simulink model "ADC_model_jitter_metaestab_v2"  (R2023b)
settings: Solver=VariableStepAuto  StartTime=0.0  StopTime=simtime  FixedStep=(1/fclk)/OSR  RelTol=1e-12
model workspace (MAT data in the model file):
  Delay_242 = [0 0 0]
  ENOB_242 = -inf
  FUNDF_242 = [nan nan]
  FUNDX_242 = [-inf -inf]
  GainError_249 = [1.75 0.02734375 2.734375]
  IMODF_242 = [nan nan]
  IMODX_242 = [nan nan]
  NoiseFloor_242 = -54.2607794062
  OIP3_242 = nan
  OffsetError_249 = [0.74921875 0.0117065429687 1.17065429687]
  SFDR_242 = inf
  SINAD_242 = -inf
  SNR_242 = -inf
  THD_242 = nan
  best_linear_fit_249 = [0.0225228416502 0.00504547332987]
  bf_dnl_249 = [0.503760731487 -0.129615618295 -0.129615618295 0.0703843817053 -0.0296156182947 -0.279615618295 0.220384381705 -0.129615618295 -0.0296156182947 0.220384381705 -0.0796156182947 -0.129615618295 -0.0296156182947 -0.129615618295 0.0703843817053 -0.0296156182947 0.170384381705 -0.229615618295 -0.0296156182947 -0.0796156182947 0.220384381705 -0.129615618295 -0.129615618295 0.0703843817053 -0.129615618295 0.170384381705 -0.0296156182947 -0.129615618295 0.0703843817053 -0.0296156182947 0.170384381705 -0.179615618295 -0.0296156182947 0.0203843817053 -0.0296156182947 -0.0296156182947 0.0703843817053 0.170384381705 0.0203843817053 -0.129615618295 0.170384381705 -0.279615618295 0.0703843817053 0.170384381705 -0.179615618295 0.120384381705 0.170384381705 -0.129615618295 -0.0296156182947 0.0703843817053 0.0703843817053 -0.129615618295 0.370384381705 -0.229615618295 0.270384381705 -0.379615618295 0.420384381705 -0.0296156182947 -0.229615618295 0.170384381705 0.0703843817053 0.170384381705 -0.0796156182947 0]
  bf_inl_249 = [0 0.503760731487 0.374145113192 0.244529494898 0.314913876603 0.285298258308 0.00568264001369 0.226067021719 0.0964514034243 0.0668357851297 0.287220166835 0.20760454854 0.0779889302457 0.048373311951 -0.0812423063437 -0.0108579246384 -0.040473542933 0.129910838772 -0.0997047795224 -0.129320397817 -0.208936016112 0.0114483655936 -0.118167252701 -0.247782870996 -0.17739848929 -0.307014107585 -0.13662972588 -0.166245344174 -0.295860962469 -0.225476580764 -0.255092199058 -0.0847078173531 -0.264323435648 -0.293939053942 -0.273554672237 -0.303170290532 -0.332785908826 -0.262401527121 -0.0920171454158 -0.0716327637105 -0.201248382005 -0.0308640002998 -0.310479618594 -0.240095236889 -0.0697108551838 -0.249326473478 -0.128942091773 0.0414422899322 -0.0881733283625 -0.117788946657 -0.0474045649518 0.0229798167535 -0.106635801541 0.263748580164 0.0341329618695 0.304517343575 -0.0750982747199 0.345286106985 0.315670488691 0.0860548703961 0.256439252101 0.326823633807 0.497208015512 0.417592397217]
  delay_242 = [0 0 0]
  ep_dnl_249 = [-8.24737104007e-15 -0.128225806452 -0.128225806452 0.0717741935484 -0.0282258064516 -0.278225806452 0.221774193548 -0.128225806452 -0.0282258064516 0.221774193548 -0.0782258064516 -0.128225806452 -0.0282258064516 -0.128225806452 0.0717741935484 -0.0282258064516 0.171774193548 -0.228225806452 -0.0282258064516 -0.0782258064516 0.221774193548 -0.128225806452 -0.128225806452 0.0717741935484 -0.128225806452 0.171774193548 -0.0282258064516 -0.128225806452 0.0717741935484 -0.0282258064516 0.171774193548 -0.178225806452 -0.0282258064516 0.0217741935484 -0.0282258064516 -0.0282258064516 0.0717741935484 0.171774193548 0.0217741935484 -0.128225806452 0.171774193548 -0.278225806452 0.0717741935484 0.171774193548 -0.178225806452 0.121774193548 0.171774193548 -0.128225806452 -0.0282258064516 0.0717741935484 0.0717741935484 -0.128225806452 0.371774193548 -0.228225806452 0.271774193548 -0.378225806452 0.421774193548 -0.0282258064516 -0.228225806452 0.171774193548 0.0717741935484 0.171774193548 -0.0782258064516 0]
  ep_inl_249 = [0 -8.24737104007e-15 -0.128225806452 -0.256451612903 -0.184677419355 -0.212903225806 -0.491129032258 -0.26935483871 -0.397580645161 -0.425806451613 -0.204032258065 -0.282258064516 -0.410483870968 -0.438709677419 -0.566935483871 -0.495161290323 -0.523387096774 -0.351612903226 -0.579838709677 -0.608064516129 -0.686290322581 -0.464516129032 -0.592741935484 -0.720967741935 -0.649193548387 -0.777419354839 -0.60564516129 -0.633870967742 -0.762096774194 -0.690322580645 -0.718548387097 -0.546774193548 -0.725 -0.753225806452 -0.731451612903 -0.759677419355 -0.787903225806 -0.716129032258 -0.54435483871 -0.522580645161 -0.650806451613 -0.479032258065 -0.757258064516 -0.685483870968 -0.513709677419 -0.691935483871 -0.570161290323 -0.398387096774 -0.526612903226 -0.554838709677 -0.483064516129 -0.411290322581 -0.539516129032 -0.167741935484 -0.395967741936 -0.124193548387 -0.502419354839 -0.0806451612903 -0.108870967742 -0.337096774194 -0.165322580645 -0.0935483870968 0.0782258064516 -2.03012210217e-14]
  nbits_249 = 6
  tcr_249(1).analog = [0.00435791015625 0.0262329101562]
  tcr_249(1).digital = 0
  tcr_249(2).analog = [0.0284204101562 0.0437329101562]
  tcr_249(2).digital = 1
  tcr_249(3).analog = [0.0502954101562 0.0634204101562]
  tcr_249(3).digital = 2
  tcr_249(4).analog = [0.0699829101562 0.0896704101562]
  tcr_249(4).digital = 3
  tcr_249(5).analog = [0.0918579101562 0.107170410156]
  tcr_249(5).digital = 4
  tcr_249(6).analog = [0.118107910156 0.124670410156]
  tcr_249(6).digital = 5
  tcr_249(7).analog = [0.133420410156 0.155295410156]
  tcr_249(7).digital = 6
  tcr_249(8).analog = [0.157482910156 0.174982910156]
  tcr_249(8).digital = 7
  tcr_249(9).analog = [0.177170410156 0.190295410156]
  tcr_249(9).digital = 8
  tcr_249(10).analog = [0.205607910156 0.218732910156]
  tcr_249(10).digital = 9
  tcr_249(11).analog = [0.231857910156 0.240607910156]
  tcr_249(11).digital = 10
  tcr_249(12).analog = [0.251545410156 0.264670410156]
  tcr_249(12).digital = 11
  tcr_249(13).analog = [0.266857910156 0.286545410156]
  tcr_249(13).digital = 12
  tcr_249(14).analog = [0.288732910156 0.306232910156]
  tcr_249(14).digital = 13
  tcr_249(15).analog = [0.308420410156 0.330295410156]
  tcr_249(15).digital = 14
  tcr_249(16).analog = [0.332482910156 0.349982910156]
  tcr_249(16).digital = 15
  tcr_249(17).analog = [0.356545410156 0.378420410156]
  tcr_249(17).digital = 16
  tcr_249(18).analog = [0.380607910156 0.393732910156]
  tcr_249(18).digital = 17
  tcr_249(19).analog = [0.400295410156 0.417795410156]
  tcr_249(19).digital = 18
  tcr_249(20).analog = [0.419982910156 0.433107910156]
  tcr_249(20).digital = 19
  tcr_249(21).analog = [0.446232910156 0.465920410156]
  tcr_249(21).digital = 20
  tcr_249(22).analog = [0.468107910156 0.485607910156]
  tcr_249(22).digital = 21
  tcr_249(23).analog = [0.487795410156 0.505295410156]
  tcr_249(23).digital = 22
  tcr_249(24).analog = [0.507482910156 0.524982910156]
  tcr_249(24).digital = 23
  tcr_249(25).analog = [0.535920410156 0.549045410156]
  tcr_249(25).digital = 24
  tcr_249(26).analog = [0.551232910156 0.575295410156]
  tcr_249(26).digital = 25
  tcr_249(27).analog = [0.577482910156 0.592795410156]
  tcr_249(27).digital = 26
  tcr_249(28).analog = [0.603732910156 0.616857910156]
  tcr_249(28).digital = 27
  tcr_249(29).analog = [0.619045410156 0.638732910156]
  tcr_249(29).digital = 28
  tcr_249(30).analog = [0.645295410156 0.662795410156]
  tcr_249(30).digital = 29
  tcr_249(31).analog = [0.664982910156 0.689045410156]
  tcr_249(31).digital = 30
  tcr_249(32).analog = [0.691232910156 0.702170410156]
  tcr_249(32).digital = 31
  tcr_249(33).analog = [0.715295410156 0.724045410156]
  tcr_249(33).digital = 32
  tcr_249(34).analog = [0.737170410156 0.750295410156]
  tcr_249(34).digital = 33
  tcr_249(35).analog = [0.756857910156 0.769982910156]
  tcr_249(35).digital = 34
  tcr_249(36).analog = [0.780920410156 0.796232910156]
  tcr_249(36).digital = 35
  tcr_249(37).analog = [0.798420410156 0.820295410156]
  tcr_249(37).digital = 36
  tcr_249(38).analog = [0.822482910156 0.846545410156]
  tcr_249(38).digital = 37
  tcr_249(39).analog = [0.848732910156 0.866232910156]
  tcr_249(39).digital = 38
  tcr_249(40).analog = [0.874982910156 0.883732910156]
  tcr_249(40).digital = 39
  tcr_249(41).analog = [0.896857910156 0.912170410156]
  tcr_249(41).digital = 40
  tcr_249(42).analog = [0.920920410156 0.931857910156]
  tcr_249(42).digital = 41
  tcr_249(43).analog = [0.934045410156 0.953732910156]
  tcr_249(43).digital = 42
  tcr_249(44).analog = [0.960295410156 0.982170410156]
  tcr_249(44).digital = 43
  tcr_249(45).analog = [0.984357910156 0.997482910156]
  tcr_249(45).digital = 44
  tcr_249(46).analog = [1.00623291016 1.02373291016]
  tcr_249(46).digital = 45
  tcr_249(47).analog = [1.03029541016 1.05217041016]
  tcr_249(47).digital = 46
  tcr_249(48).analog = [1.05435791016 1.06967041016]
  tcr_249(48).digital = 47
  tcr_249(49).analog = [1.07623291016 1.08935791016]
  tcr_249(49).digital = 48
  tcr_249(50).analog = [1.10029541016 1.11779541016]
  tcr_249(50).digital = 49
  tcr_249(51).analog = [1.11998291016 1.13967041016]
  tcr_249(51).digital = 50
  tcr_249(52).analog = [1.14623291016 1.15935791016]
  tcr_249(52).digital = 51
  tcr_249(53).analog = [1.16592041016 1.19217041016]
  tcr_249(53).digital = 52
  tcr_249(54).analog = [1.19435791016 1.20967041016]
  tcr_249(54).digital = 53
  tcr_249(55).analog = [1.21185791016 1.23810791016]
  tcr_249(55).digital = 54
  tcr_249(56).analog = [1.24029541016 1.24904541016]
  tcr_249(56).digital = 55
  tcr_249(57).analog = [1.25779541016 1.27967041016]
  tcr_249(57).digital = 56
  tcr_249(58).analog = [1.29060791016 1.30592041016]
  tcr_249(58).digital = 57
  tcr_249(59).analog = [1.30810791016 1.32123291016]
  tcr_249(59).digital = 58
  tcr_249(60).analog = [1.32779541016 1.34748291016]
  tcr_249(60).digital = 59
  tcr_249(61).analog = [1.35404541016 1.37154541016]
  tcr_249(61).digital = 60
  tcr_249(62).analog = [1.37810791016 1.39998291016]
  tcr_249(62).digital = 61
  tcr_249(63).analog = [1.40217041016 1.41529541016]
  tcr_249(63).digital = 62
  tcr_249(64).analog = [1.42842041016 1.74998291016]
  tcr_249(64).digital = 63
  v_high_249 = 1.4
  v_low_249 = 0
values from neighbouring files (symbols this model uses):
  Ah2 = 0    [dynamic_charac_defaultvalues.mat]    (also in static_charac_defaultvalues.mat = 4.24264068712e-05)
  Ah3 = 0    [dynamic_charac_defaultvalues.mat]    (also in static_charac_defaultvalues.mat = 0.000707106781187)
  Ah4 = 0    [dynamic_charac_defaultvalues.mat]    (also in static_charac_defaultvalues.mat = 4.24264068712e-05)
  Ah5 = 0    [dynamic_charac_defaultvalues.mat]    (also in static_charac_defaultvalues.mat = 0.000141421356237)
  Ain = 0.45    [dynamic_charac_defaultvalues.mat]    (also in static_charac_defaultvalues.mat)
  B = 8    [dynamic_charac_defaultvalues.mat]    (also in static_charac_defaultvalues.mat)
  clock_type = 2    [dynamic_charac_defaultvalues.mat]    (also in static_charac_defaultvalues.mat)
  comparator_noise_state = 1    [dynamic_charac_defaultvalues.mat]    (also in static_charac_defaultvalues.mat)
  const = 0.8    [dynamic_charac_defaultvalues.mat]    (also in static_charac_defaultvalues.mat)
  e1 = 0    [dynamic_charac_defaultvalues.mat]    (also in static_charac_defaultvalues.mat)
  e2 = 0    [dynamic_charac_defaultvalues.mat]    (also in static_charac_defaultvalues.mat)
  e3 = 0    [dynamic_charac_defaultvalues.mat]    (also in static_charac_defaultvalues.mat)
  eoff = 0    [dynamic_charac_defaultvalues.mat]    (also in static_charac_defaultvalues.mat)
  fclk = 100000000    [dynamic_charac_defaultvalues.mat]    (also in static_charac_defaultvalues.mat)
  fin = 38337.7075195    [dynamic_charac_defaultvalues.mat]    (also in static_charac_defaultvalues.mat = 1)
  final_value = 1.25    [dynamic_charac_defaultvalues.mat]    (also in static_charac_defaultvalues.mat)
  FS = 1    [dynamic_charac_defaultvalues.mat]    (also in static_charac_defaultvalues.mat)
  fs = 390625    [dynamic_charac_defaultvalues.mat]    (also in static_charac_defaultvalues.mat = 1)
  initial_value = 0    [dynamic_charac_defaultvalues.mat]    (also in static_charac_defaultvalues.mat)
  input_type = 3    [dynamic_charac_defaultvalues.mat]    (also in static_charac_defaultvalues.mat = 1)
  M = 1280    [dynamic_charac_defaultvalues.mat]    (also in static_charac_defaultvalues.mat)
  mean_alpha = 0    [dynamic_charac_defaultvalues.mat]    (also in static_charac_defaultvalues.mat)
  mean_beta = 0.5    [dynamic_charac_defaultvalues.mat]    (also in static_charac_defaultvalues.mat)
  noise_Vrms = 0.0001    [dynamic_charac_defaultvalues.mat]    (also in static_charac_defaultvalues.mat)
  OSR = 2    [dynamic_charac_defaultvalues.mat]    (also in static_charac_defaultvalues.mat)
  ramp_noise_state = 1    [dynamic_charac_defaultvalues.mat]    (also in static_charac_defaultvalues.mat)
  SEED1 = 15581    [dynamic_charac_defaultvalues.mat]    (also in static_charac_defaultvalues.mat = 13575)
  SEED2 = 7150    [dynamic_charac_defaultvalues.mat]    (also in static_charac_defaultvalues.mat = 7577)
  sigma_alpha = 1e-10    [dynamic_charac_defaultvalues.mat]    (also in static_charac_defaultvalues.mat)
  sigma_beta = 1e-10    [dynamic_charac_defaultvalues.mat]    (also in static_charac_defaultvalues.mat)
  tau = 1e-16    [dynamic_charac_defaultvalues.mat]    (also in static_charac_defaultvalues.mat = 1e-11)
  tphase = 1e-08    [dynamic_charac_defaultvalues.mat]    (also in static_charac_defaultvalues.mat)
  Ts = 1e-08    [dynamic_charac_defaultvalues.mat]    (also in static_charac_defaultvalues.mat)
  Vnoise_comparator = 1e-10    [dynamic_charac_defaultvalues.mat]    (also in static_charac_defaultvalues.mat)
  Vnoise_ramp = 1e-10    [dynamic_charac_defaultvalues.mat]    (also in static_charac_defaultvalues.mat)
  Vof_comparator = 0    [dynamic_charac_defaultvalues.mat]    (also in static_charac_defaultvalues.mat)
libraries: simulink x4, simulink_extras x2, msbAdcFoundation x1
settings Model: SimulationMode=accelerator  Creator=mario  LastModifiedBy=mario
settings SolverCC: ZeroCrossAlgorithm=Adaptive
settings DataIOCC: SaveOutput=off  SignalLogging=off  DSMLogging=off  SaveTime=off

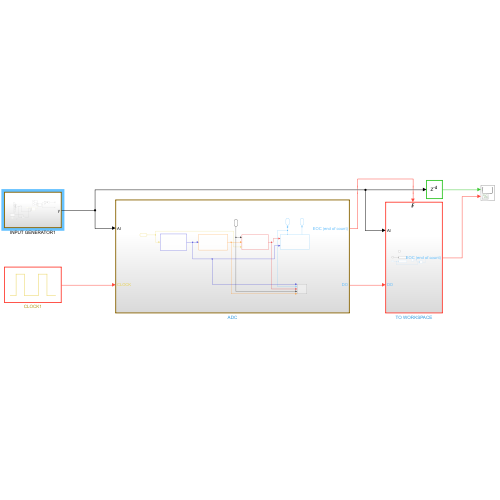
[thumbnail: Simulink's stored preview of the top-level diagram]
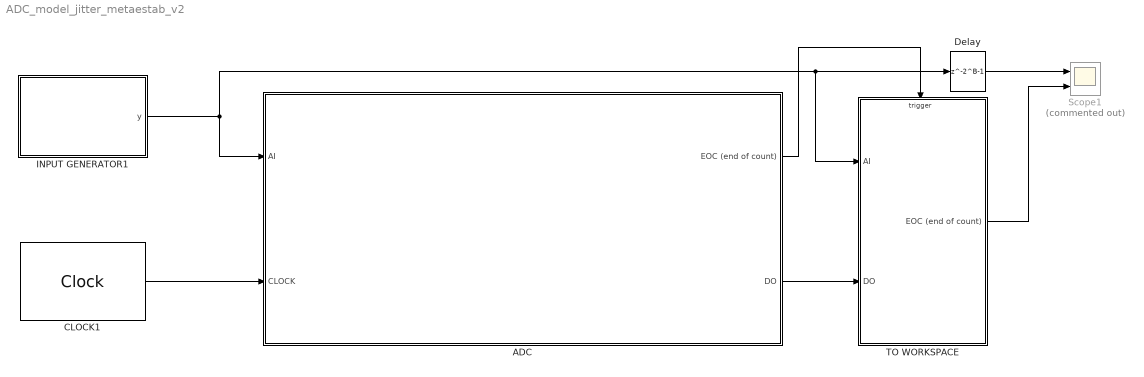
== system ADC_model_jitter_metaestab_v2 ==
  ADC : Subsystem
  CLOCK1 : simulink_extras/Flip Flops/Clock  period=1/fclk
  Delay : Delay  DelayLength=2^B-1  InitialCondition=0  SampleTime=1/fclk
  INPUT GENERATOR1 : Subsystem
  Scope1 : Scope  Commented=on  NumInputPorts=2
  TO WORKSPACE : Subsystem
  wires:
  ADC/1(EOC (end of count)) -> TO WORKSPACE/Trigger
  INPUT GENERATOR1/1(y) -> ADC/1(AI), TO WORKSPACE/1(AI), Delay/1
  TO WORKSPACE/1(EOC (end of count)) -> Scope1/2
  Delay/1 -> Scope1/1
  CLOCK1/1 -> ADC/2(CLOCK)
  ADC/2(DO) -> TO WORKSPACE/2(DO)

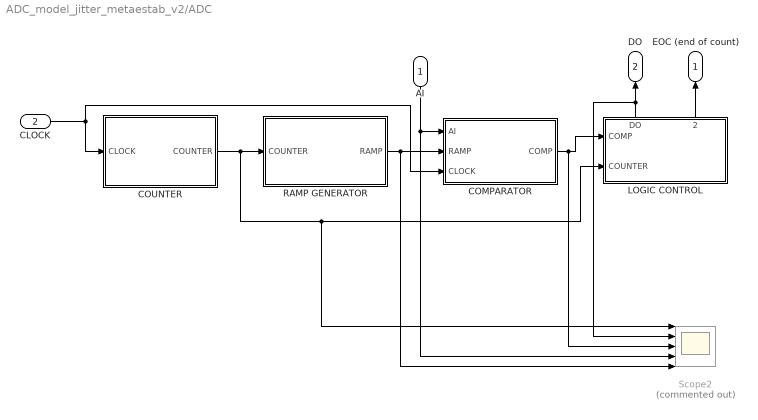
== system ADC_model_jitter_metaestab_v2/ADC ==
  AI : Inport
  CLOCK : Inport  Port=2
  COMPARATOR : Subsystem
  COUNTER : Subsystem
  LOGIC CONTROL : Subsystem
      settings: PortSchema="{\"entries\":[{\"content\":{\"sides\":[{\"content\":{},\"type\":\"ConnectorPlacement.EquallySpacedRectSide\",\"uuid\":\"4dac15f4-60b2-47ff-be01-608d4a6ba830\"},{\"content\":{\"connectorIds\":[\"Out1\",\"Out2\"],\"side\":\"RIGHT\"},\"type\":\"ConnectorPlacement.EquallySpacedRectSide\",\"uuid\":\"a37273df-03c3-4eb4-bc46-6efba4b33bab\"},{\"content\":{\"connectorIds\":[\"In1\",\"In2\"],\"side\":\"TOP\"},\"type\":\"ConnectorPlacement.EquallySpacedRectSide\",\"uuid\":\"d6687def-ae8a-4e2e-b37c-f0a7dff58a2e\"}]},\"type\":\"ConnectorPlacement.EquallySpacedConnector\",\"uuid\":\"dcf8488a-4d66-42cb-896c-32122c97ab88\"}],\"packageUris\":[\"http://schema.mathworks.com/mf0/Connector/R2020b\"],\"version\":\"1.0\"}"
  RAMP GENERATOR : Subsystem
  Scope2 : Scope  Commented=on  NumInputPorts=5
  EOC (end of count) : Outport
  DO : Outport  Port=2
  wires:
  CLOCK/1 -> COMPARATOR/3(CLOCK), COUNTER/1(CLOCK)
  AI/1 -> Scope2/4, COMPARATOR/1(AI)
  LOGIC CONTROL/1(DO) -> Scope2/2, DO/1
  LOGIC CONTROL/2(EOC (end of count)) -> EOC (end of count)/1
  COMPARATOR/1(COMP) -> Scope2/3, LOGIC CONTROL/2(COMP)
  COUNTER/1(COUNTER) -> Scope2/1, LOGIC CONTROL/1(COUNTER), RAMP GENERATOR/1(COUNTER)
  RAMP GENERATOR/1(RAMP) -> Scope2/5, COMPARATOR/2(RAMP)

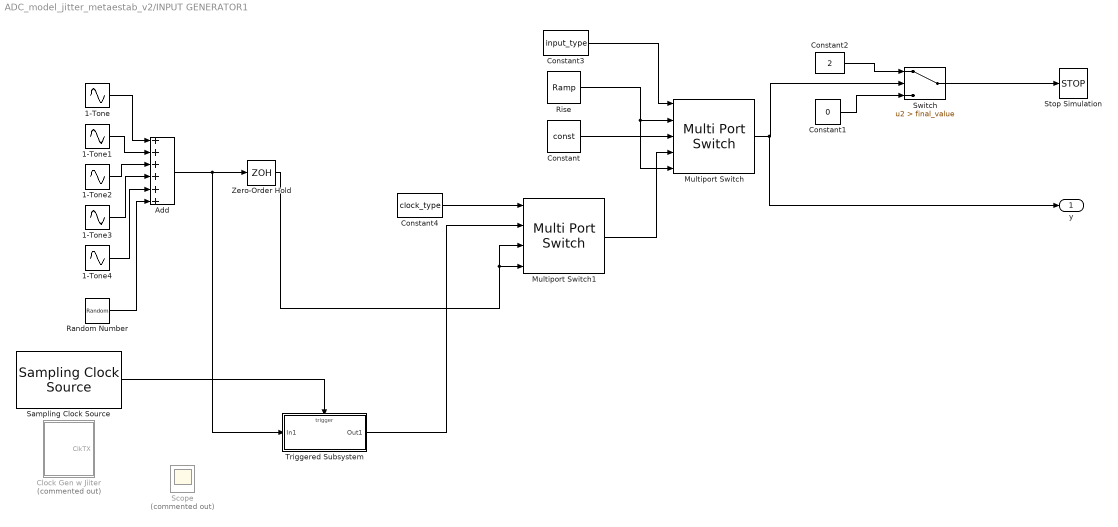
== system ADC_model_jitter_metaestab_v2/INPUT GENERATOR1 ==
  1-Tone : Sin  Amplitude=Ain  Bias=FS/2  Frequency=2 * pi * fin  SampleTime=0
  1-Tone1 : Sin  Amplitude=Ah2  Frequency=2 * pi * 2*fin  Phase=2*pi*randn  SampleTime=0
  1-Tone2 : Sin  Amplitude=Ah3  Frequency=2 * pi * 3*fin  Phase=2*pi*randn  SampleTime=0
  1-Tone3 : Sin  Amplitude=Ah4  Frequency=2 * pi * 4*fin  Phase=2*pi*randn  SampleTime=0
  1-Tone4 : Sin  Amplitude=Ah5  Frequency=2 * pi * 5*fin  Phase=2*pi*randn  SampleTime=0
  Add : Sum  Inputs=++++++
  Clock Gen w Jiiter : Subsystem  Commented=on
  Constant : Constant  Value=const
  Constant1 : Constant  Value=0
  Constant2 : Constant  Value=2
  Constant3 : Constant  Value=input_type
  Constant4 : Constant  Value=clock_type
  Multiport Switch : MultiPortSwitch  DataPortForDefault=Additional data port  DiagnosticForDefault=None  SaturateOnIntegerOverflow=off  InputSameDT=off
  Multiport Switch1 : MultiPortSwitch  Inputs=2  DataPortForDefault=Additional data port  DiagnosticForDefault=None  SaturateOnIntegerOverflow=off  InputSameDT=off
  Random Number : RandomNumber  Variance=noise_Vrms^2  SampleTime=0
  Rise : simulink/Sources/Ramp  slope=FS/((1/fclk)*(2^B)*(M))  start=0  InitialOutput=initial_value
  Sampling Clock Source : msbAdcFoundation/Sampling Clock Source  Freq=fs  Min=0  Max=1  RmsJitt=ap_jitter  CustomSeed=off  Seed=0  CustomInitialOutput=off  InitialOutput=1  ExtraBuffer=off  NBuffer=50
      settings: SignalType=Square wave
  Scope : Scope  Commented=on  NumInputPorts=2
  Stop Simulation : Stop
  Switch : Switch  Criteria=u2 > Threshold  Threshold=final_value  SaturateOnIntegerOverflow=off  InputSameDT=off
  Triggered Subsystem : Subsystem  TreatAsAtomicUnit=on
  Zero-Order Hold : ZeroOrderHold  SampleTime=1/fs
  y : Outport
  wires:
  Zero-Order Hold/1 -> Multiport Switch1/3, Multiport Switch1/4
  1-Tone/1 -> Add/1
  1-Tone1/1 -> Add/2
  Random Number/1 -> Add/6
  1-Tone4/1 -> Add/5
  1-Tone3/1 -> Add/4
  1-Tone2/1 -> Add/3
  Add/1 -> Triggered Subsystem/1(In1), Zero-Order Hold/1
  Constant4/1 -> Multiport Switch1/1
  Triggered Subsystem/1(Out1) -> Multiport Switch1/2
  Multiport Switch1/1 -> Multiport Switch/4
  Multiport Switch/1 -> Switch/2, y/1
  Rise/1 -> Multiport Switch/5, Multiport Switch/2
  Constant3/1 -> Multiport Switch/1
  Constant/1 -> Multiport Switch/3
  Switch/1 -> Stop Simulation/1
  Constant1/1 -> Switch/3
  Constant2/1 -> Switch/1
  Sampling Clock Source/1 -> Triggered Subsystem/Trigger

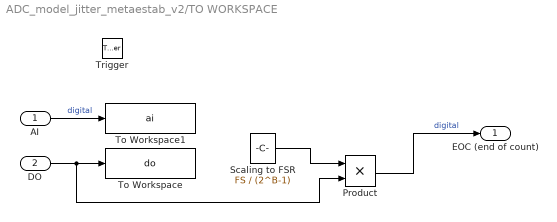
== system ADC_model_jitter_metaestab_v2/TO WORKSPACE ==
  AI : Inport
  DO : Inport  Port=2
  Trigger : TriggerPort  VariantControl=Variant  ZeroCross=off  PortDimensions=1
  Product : Product
  Scaling to FSR : Constant  Value=FS / (2^B-1)
  To Workspace : ToWorkspace  VariableName=do  SaveFormat=Structure With Time  SampleTime=-1
      settings: Save2DSignal=2-D array (concatenate along first dimension)
  To Workspace1 : ToWorkspace  VariableName=ai  SaveFormat=Structure  SampleTime=-1
      settings: Save2DSignal=2-D array (concatenate along first dimension)
  EOC (end of count) : Outport
  wires:
  DO/1 -> Product/2, To Workspace/1
  Product/1 -> EOC (end of count)/1  "digital"
  AI/1 -> To Workspace1/1  "digital"
  Scaling to FSR/1 -> Product/1

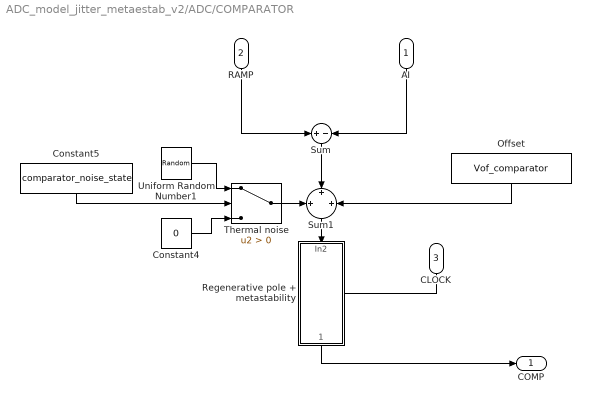
== system ADC_model_jitter_metaestab_v2/ADC/COMPARATOR ==
  AI : Inport
  RAMP : Inport  Port=2
  CLOCK : Inport  Port=3
  Constant4 : Constant  Value=0
  Constant5 : Constant  Value=comparator_noise_state
  Offset : Constant  Value=Vof_comparator
  Regenerative pole + metastability : Subsystem  TreatAsAtomicUnit=on
  Sum : Sum  Inputs=+|-
  Sum1 : Sum  Inputs=+|+|+
  Thermal noise : Switch  Criteria=u2 > Threshold  SaturateOnIntegerOverflow=off  InputSameDT=off
  Uniform Random Number1 : UniformRandomNumber  Minimum=-Vnoise_comparator  Maximum=Vnoise_comparator  Seed=SEED2  SampleTime=1/(2*fclk)
  COMP : Outport
  wires:
  Regenerative pole + metastability/1(OUT COMP) -> COMP/1
  Sum/1 -> Sum1/2
  Uniform Random Number1/1 -> Thermal noise/1
  Thermal noise/1 -> Sum1/1
  Constant4/1 -> Thermal noise/3
  Constant5/1 -> Thermal noise/2
  Offset/1 -> Sum1/3
  AI/1 -> Sum/2
  RAMP/1 -> Sum/1
  CLOCK/1 -> Regenerative pole + metastability/Trigger
  Sum1/1 -> Regenerative pole + metastability/1(In2)

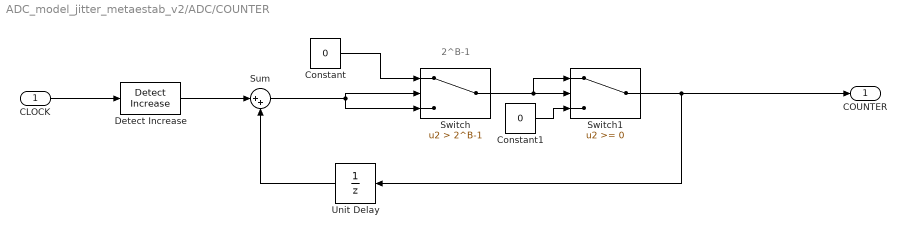
== system ADC_model_jitter_metaestab_v2/ADC/COUNTER ==
  note: 2^B-1
  CLOCK : Inport
  Constant : Constant  Value=0
  Constant1 : Constant  Value=0
  Detect Increase : simulink/Logic and Bit Operations/Detect Increase  vinit=0.0  OutDataTypeStr=boolean
  Sum : Sum  Inputs=|++
  Switch : Switch  Criteria=u2 > Threshold  Threshold=2^B-1  SaturateOnIntegerOverflow=off  InputSameDT=off
  Switch1 : Switch  SaturateOnIntegerOverflow=off  InputSameDT=off
  Unit Delay : UnitDelay  InitialCondition=-1  SampleTime=-1  HasFrameUpgradeWarning=on
  COUNTER : Outport
  wires:
  Sum/1 -> Switch/2, Switch/3
  Constant/1 -> Switch/1
  Unit Delay/1 -> Sum/2
  CLOCK/1 -> Detect Increase/1
  Detect Increase/1 -> Sum/1
  Switch1/1 -> Unit Delay/1, COUNTER/1
  Switch/1 -> Switch1/1, Switch1/2
  Constant1/1 -> Switch1/3

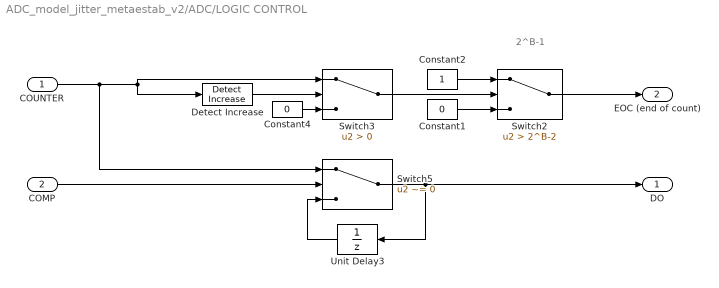
== system ADC_model_jitter_metaestab_v2/ADC/LOGIC CONTROL ==
  note: 2^B-1
  COUNTER : Inport
  COMP : Inport  Port=2
  Constant1 : Constant  Value=0
  Constant2 : Constant
  Constant4 : Constant  Value=0
  Detect Increase : simulink/Logic and Bit Operations/Detect Increase  vinit=0.0  OutDataTypeStr=boolean
  Switch2 : Switch  Criteria=u2 > Threshold  Threshold=2^B-2  SaturateOnIntegerOverflow=off  InputSameDT=off
  Switch3 : Switch  Criteria=u2 > Threshold  SaturateOnIntegerOverflow=off  InputSameDT=off
  Switch5 : Switch  Criteria=u2 ~= 0  SaturateOnIntegerOverflow=off  InputSameDT=off
  Unit Delay3 : UnitDelay  SampleTime=-1  HasFrameUpgradeWarning=on
  DO : Outport
  EOC (end of count) : Outport  Port=2
  wires:
  Constant1/1 -> Switch2/3
  Constant2/1 -> Switch2/1
  Detect Increase/1 -> Switch3/2
  COUNTER/1 -> Switch3/1, Detect Increase/1, Switch5/1
  Switch3/1 -> Switch2/2
  Constant4/1 -> Switch3/3
  COMP/1 -> Switch5/2
  Switch2/1 -> EOC (end of count)/1
  Switch5/1 -> Unit Delay3/1, DO/1
  Unit Delay3/1 -> Switch5/3

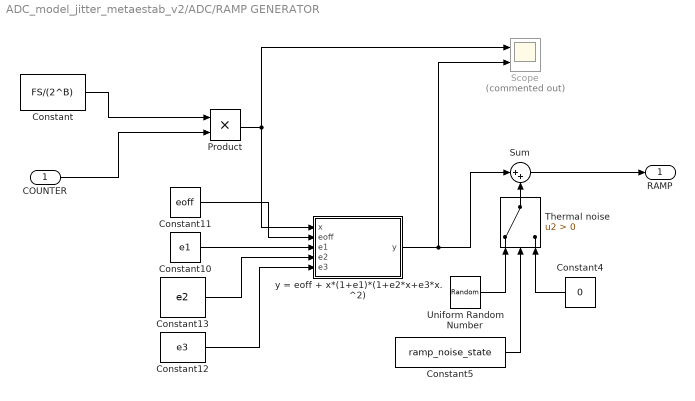
== system ADC_model_jitter_metaestab_v2/ADC/RAMP GENERATOR ==
  COUNTER : Inport
  Constant : Constant  Value=FS/(2^B)
  Constant10 : Constant  Value=e1
  Constant11 : Constant  Value=eoff
  Constant12 : Constant  Value=e3
  Constant13 : Constant  Value=e2
  Constant4 : Constant  Value=0
  Constant5 : Constant  Value=ramp_noise_state
  Product : Product
  Scope : Scope  Commented=on  NumInputPorts=2
  Sum : Sum  Inputs=|++
  Thermal noise : Switch  Criteria=u2 > Threshold  SaturateOnIntegerOverflow=off  InputSameDT=off
  Uniform Random Number : UniformRandomNumber  Minimum=-Vnoise_ramp  Maximum=Vnoise_ramp  Seed=SEED1  SampleTime=1/(2*fclk)
  y = eoff + x*(1+e1)*(1+e2*x+e3*x.^2) : MATLAB Function
  RAMP : Outport
  wires:
  COUNTER/1 -> Product/2
  Constant/1 -> Product/1
  Constant5/1 -> Thermal noise/2
  Constant4/1 -> Thermal noise/3
  Uniform Random Number/1 -> Thermal noise/1
  Thermal noise/1 -> Sum/2
  Constant10/1 -> y = eoff + x*(1+e1)*(1+e2*x+e3*x.^2)/3(e1)
  Constant11/1 -> y = eoff + x*(1+e1)*(1+e2*x+e3*x.^2)/2(eoff)
  Constant12/1 -> y = eoff + x*(1+e1)*(1+e2*x+e3*x.^2)/5(e3)
  Constant13/1 -> y = eoff + x*(1+e1)*(1+e2*x+e3*x.^2)/4(e2)
  Sum/1 -> RAMP/1
  y = eoff + x*(1+e1)*(1+e2*x+e3*x.^2)/1(y) -> Scope/2, Sum/1
  Product/1 -> Scope/1, y = eoff + x*(1+e1)*(1+e2*x+e3*x.^2)/1(x)

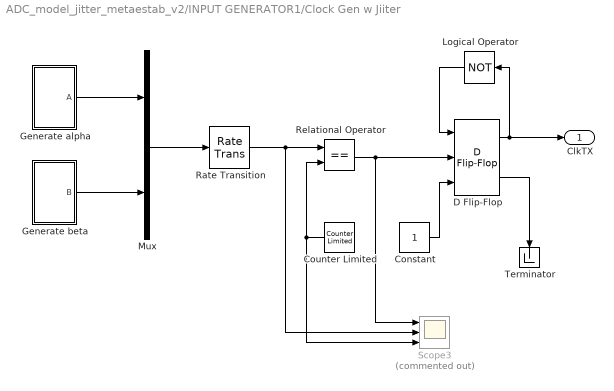
== system ADC_model_jitter_metaestab_v2/INPUT GENERATOR1/Clock Gen w Jiiter ==
  Constant : Constant
  Counter Limited : simulink/Sources/Counter Limited  uplimit=OSR-1  tsamp=Ts/OSR
  D Flip-Flop : simulink_extras/Flip Flops/D Flip-Flop
  Generate alpha : Subsystem
  Generate beta : Subsystem
  Logical Operator : Logic  Operator=NOT  Inputs=1  AllPortsSameDT=off  OutDataTypeStr=boolean
  Mux : Mux  Inputs=2
  Rate Transition : RateTransition  OutPortSampleTime=Ts/OSR
  Relational Operator : RelationalOperator  Operator===  OutDataTypeStr=boolean  RndMeth=Simplest  InputSameDT=off
  Scope3 : Scope  Commented=on  NumInputPorts=3
  Terminator : Terminator
  ClkTX : Outport
  wires:
  Rate Transition/1 -> Relational Operator/1, Scope3/2
  D Flip-Flop/1 -> Logical Operator/1, ClkTX/1
  Generate alpha/1(A) -> Mux/1
  Constant/1 -> D Flip-Flop/3
  Mux/1 -> Rate Transition/1
  Generate beta/1(B) -> Mux/2
  Logical Operator/1 -> D Flip-Flop/1
  Counter Limited/1 -> Relational Operator/2, Scope3/3
  Relational Operator/1 -> D Flip-Flop/2, Scope3/1
  D Flip-Flop/2 -> Terminator/1

== system ADC_model_jitter_metaestab_v2/INPUT GENERATOR1/Triggered Subsystem ==
  In1 : Inport
  Trigger : TriggerPort  VariantControl=(inherit)
  Out1 : Outport
  wires:
  In1/1 -> Out1/1

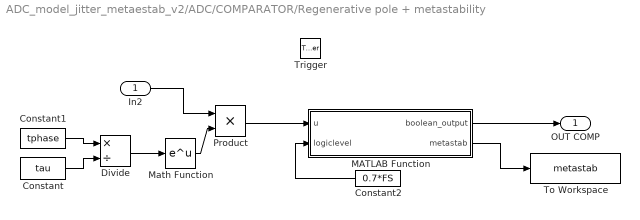
== system ADC_model_jitter_metaestab_v2/ADC/COMPARATOR/Regenerative pole + metastability ==
  In2 : Inport
  Trigger : TriggerPort  VariantControl=(inherit)
  Constant : Constant  Value=tau
  Constant1 : Constant  Value=tphase
  Constant2 : Constant  Value=0.7*FS
  Divide : Product  Inputs=*/
  MATLAB Function : MATLAB Function  TreatAsAtomicUnit=on
  Math Function : Math
  Product : Product
  To Workspace : ToWorkspace  VariableName=metastab  SampleTime=-1
  OUT COMP : Outport
  wires:
  MATLAB Function/1(boolean_output) -> OUT COMP/1
  Product/1 -> MATLAB Function/1(u)
  Constant/1 -> Divide/2
  Divide/1 -> Math Function/1
  Constant1/1 -> Divide/1
  Math Function/1 -> Product/2
  In2/1 -> Product/1
  MATLAB Function/2(metastab) -> To Workspace/1
  Constant2/1 -> MATLAB Function/2(logiclevel)

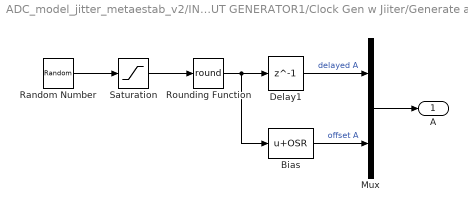
== system ADC_model_jitter_metaestab_v2/INPUT GENERATOR1/Clock Gen w Jiiter/Generate alpha ==
  Bias : Bias  Bias=OSR  SaturateOnIntegerOverflow=off
  Delay1 : Delay  DelayLength=1  SampleTime=Ts
  Mux : Mux  Inputs=2
  Random Number : RandomNumber  Mean=mean_alpha*OSR  Variance=(sigma_alpha/Ts)*OSR  Seed=SEED1  SampleTime=Ts
  Rounding Function : Rounding  Operator=round
  Saturation : Saturate  UpperLimit=(mean_alpha+2*sigma_alpha/Ts)*OSR  LowerLimit=(mean_alpha-2*sigma_alpha/Ts)*OSR
  A : Outport
  wires:
  Saturation/1 -> Rounding Function/1
  Random Number/1 -> Saturation/1
  Mux/1 -> A/1
  Bias/1 -> Mux/2  "offset A"
  Delay1/1 -> Mux/1  "delayed A"
  Rounding Function/1 -> Delay1/1, Bias/1

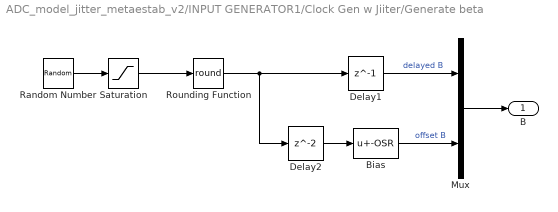
== system ADC_model_jitter_metaestab_v2/INPUT GENERATOR1/Clock Gen w Jiiter/Generate beta ==
  Bias : Bias  Bias=-OSR  SaturateOnIntegerOverflow=off
  Delay1 : Delay  DelayLength=1  SampleTime=Ts
  Delay2 : Delay  SampleTime=Ts
  Mux : Mux  Inputs=2
  Random Number : RandomNumber  Mean=mean_beta*OSR  Variance=sigma_beta/Ts*OSR  Seed=2342  SampleTime=Ts
  Rounding Function : Rounding  Operator=round
  Saturation : Saturate  UpperLimit=(mean_beta+2*sigma_beta/Ts)*OSR  LowerLimit=(mean_beta-2*sigma_beta/Ts)*OSR
  B : Outport
  wires:
  Saturation/1 -> Rounding Function/1
  Random Number/1 -> Saturation/1
  Delay2/1 -> Bias/1
  Bias/1 -> Mux/2  "offset B"
  Rounding Function/1 -> Delay1/1, Delay2/1
  Mux/1 -> B/1
  Delay1/1 -> Mux/1  "delayed B"

== matlab function ADC_model_jitter_metaestab_v2/ADC/COMPARATOR/Regenerative pole + metastability/MATLAB Function ==
  data: u input; boolean_output output; logiclevel input; metastab output
function [boolean_output, metastab] = fcn(u, logiclevel)

if u >= logiclevel
    boolean_output = 0;
    metastab = 0;
elseif u <= -logiclevel
    boolean_output = 1;
    metastab = 0;
else
    boolean_output = 1;
    metastab = 1;
end

== matlab function ADC_model_jitter_metaestab_v2/ADC/RAMP GENERATOR/y = eoff + x*(1+e1)*(1+e2*x+e3*x.^2) ==
  data: x input; y output; eoff input; e1 input; e2 input; e3 input
function y = fcn(x,eoff, e1, e2, e3)

y = eoff + x*(1+e1)*(1+e2*x+e3*x.^2);
